simulink model "nexus_block"  (R2024b)
settings: Solver=ode4  StartTime=0.0  StopTime=5  FixedStep=0.001  RelTol=1e-3  AbsTol=1e-6
values from neighbouring files (symbols this model uses):
  Acf = [Acf zeros(3,3); zeros(3,3) Acf]    [nexus_fsm.m]
  Adc = [0 1 zeros(1,10); -wc^2 -2*zij(1,1)*wc zeros(1,10) ... (first row only)    [nexus_cryo.m]
  Adg = [Adg zeros(2,2); zeros(2,2) Adg]    [nexus_gs.m]
  Ads = [-wn]    [nexus_acsnoise.m]
  Adw = [Adr_r,zeros(4,8); zeros(4,4) Adr_a zeros(4,4); zeros(4,8) Adr_t]    [nexus_rwa.m]
  Bca = Bca*Tsel*[P' zeros(3,5); zeros(3,3) P' zeros(3,2); zeros(3,6) P'*H]    [nexus_acsloop.m]
  Bcf = [Bcf zeros(3,1); zeros(3,1) Bcf]    [nexus_fsm.m]
  Bdc = [0 1 0 1 0 1 0 1 0 1 0 1]'    [nexus_cryo.m]
  Bdg = [Bdg [0 0]';[0 0]' Bdg]    [nexus_gs.m]
  Bds = [1]'    [nexus_acsnoise.m]
  Bdw = [Bdr_r ; Bdr_a ; Bdr_t]    [nexus_rwa.m]
  Cca = (-1)*P*Cca    [nexus_acsloop.m]
  Ccf = [Ccf zeros(1,3); zeros(1,3) Ccf]    [nexus_fsm.m]
  Cdc = [       zeros(1,6) 0 kij(2,1) 0 kij(2,2) 0 kij(2,3) ... (first row only)    [nexus_cryo.m]
  Cdg = a2r*[Cdg [0 0]; [0 0] Cdg]    [nexus_gs.m]
  Cds = Kn*[wn]    [nexus_acsnoise.m]
  Cdw = [Cdr_r zeros(1,8); Cdr_r zeros(1,8); zeros(1,4) Cdr_a zeros(1,4) ... (first row only)    [nexus_rwa.m]
  Dca = (-1)*P*Dca*Tsel*[P' zeros(3,5); zeros(3,3) P' zeros(3,2); zeros(3,6) P'*H]    [nexus_acsloop.m]
  dcdu = inv(m2micron)*[dcdupmseg1 dcdupmseg2 dcdupmseg3 dcdusm dcduim]    [nexus_optics.m]
  Dcf = [Dcf 0; 0 Dcf]    [nexus_fsm.m]
  Ddc = [zeros(3,1)]    [nexus_cryo.m]
  Ddg = a2r*zeros(2,2)    [nexus_gs.m]
  Dds = [0]    [nexus_acsnoise.m]
  Ddw = [zeros(6,1)]    [nexus_rwa.m]
  dt = 1/(20*wc/2/pi)    [nexus_cryo.m]    (also in nexus_perf.m = 0.001)
  dwdu = inv(m2nm)*dwdu    [nexus_optics.m]    (also in nexus_perf.m = dwdu(1:nray,1:ndof))
  Kfsm = mm2m*dcdu(:,97:98)    [nexus_optics.m]
  m2micron = 1e6    (= 1000000)    [nexus_optics.m]
  m2nm = 1e9    (= 1000000000)    [nexus_optics.m]
  psc = mean(abs([sourcerot(1,1) sourcerot(2,2)]))    [nexus_optics.m]
  Seed = round(1e5*rand(10,1))    [nexus_perf.m]
undefined symbols (not defined in the file or in its folder): Aca, Ap, Bp, Cp, Dp, R1, R2, R3, R4
libraries: simulink x10, dspstat3 x2
settings Model: Creator=June  LastModifiedBy=June
settings SolverCC: AutoScaleAbsTol=off
settings DataIOCC: SaveFormat=Array  SignalLoggingSaveFormat=ModelDataLogs  ReturnWorkspaceOutputs=off
settings OptimizationCC: BlockReduction=off  BooleanDataType=off  ZeroExternalMemoryAtStartup=off  ZeroInternalMemoryAtStartup=off  InitFltsAndDblsToZero=on  LifeSpan=inf
settings DebuggingCC: SaveWithParameterizedLinksMsg=none  UnderspecifiedInitializationDetection=Classic  MergeDetectMultiDrivingBlocksExec=none  SignalResolutionControl=TryResolveAllWithWarning  MultiTaskDSMMsg=warning  MultiTaskCondExecSysMsg=none  FcnCallInpInsideContextMsg=warning  UnconnectedInputMsg=warning  UnconnectedOutputMsg=warning  UnconnectedLineMsg=warning  SFUnexpectedBacktrackingDiag=warning  SFNoUnconditionalDefaultTransitionDiag=warning  SFExecutionAtInitializationDiag=none  ArithmeticOperatorsInVariantConditions=warning
settings HardwareCC: ProdBitPerPointer=32  ProdBitPerSizeT=32  ProdBitPerPtrDiffT=32  ProdLargestAtomicFloat=None  ProdIntDivRoundTo=Undefined  ProdEndianess=Unspecified  ProdWordSize=32  ProdHWDeviceType=32-bit Generic  TargetBitPerPointer=64  TargetBitPerSizeT=64  TargetBitPerPtrDiffT=64  TargetLongLongMode=on  TargetIntDivRoundTo=Zero  TargetEndianess=LittleEndian  TargetWordSize=64  TargetHWDeviceType=MATLAB Host  ProdEqTarget=off
settings ModelReferenceCC: PropagateSignalLabelsOutOfModel=off
settings RTWCC: TargetLang=C++  GPUComputeCapability=3.5
settings CodeAppCC: ForceParamTrailComments=on  StateflowObjectComments=on  MATLABSourceComments=on
settings GRTTargetCC: TargetFcnLib=ansi_tfl_tmw.mat  TargetLangStandard=C++11 (ISO)  ModelReferenceCompliant=off  CodeInterfacePackaging=C++ class  MultiInstanceErrorCode=Warning
settings ConfigComp: CovMetricSettings=dw  CovSaveCumulativeToWorkspaceVar=on  CovSaveSingleToWorkspaceVar=on

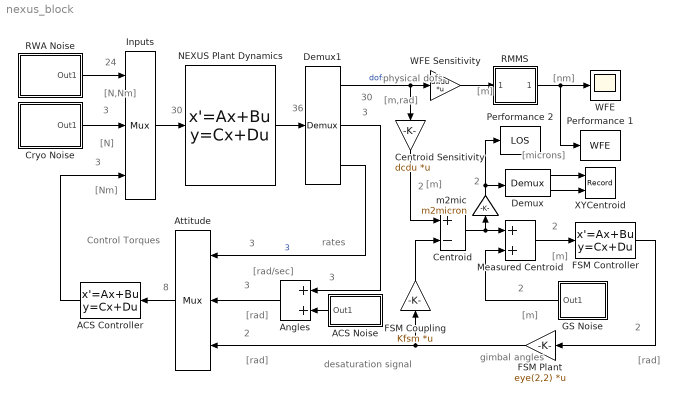
== system nexus_block ==
  note: 24
  note: 3
  note: 30
  note: 30
  note: 2
  note: 2
  note: 3
  note: 3
  note: 2
  note: 2
  note: gimbal
      | angles
  note: 36
  note: Control
      | Torques
  note: physical
      |  dofs
  note: rates
  note: 3
  note: 3
  note: 2
  note: 8
  note: desaturation signal
  note: [rad]
  note: [m,rad]
  note: [Nm]
  note: [rad/sec]
  note: [rad]
  note: [rad]
  note: [m]
  note: [m]
  note: [N,Nm]
  note: [N]
  note: [nm]
  note: [m]
  note: [microns]
  note: [m]
  note: 2
  note: 3
  ACS Controller : StateSpace  A=Aca  B=Bca  C=Cca  D=Dca  InitialCondition=0
  ACS Noise : Subsystem
  Angles : Sum  InputSameDT=on  SaturateOnIntegerOverflow=on  OutDataTypeStr=Inherit: Same as first input
  Attitude : Mux  Inputs=3
  Centroid : Sum  Inputs=+-  InputSameDT=on  SaturateOnIntegerOverflow=on  OutDataTypeStr=Inherit: Same as first input
  Centroid Sensitivity : Gain  Gain=dcdu  Multiplication=Matrix(K*u)  SaturateOnIntegerOverflow=on  OutDataTypeStr=Inherit: Same as input  ParamDataTypeStr=Inherit: Same as input
  Cryo Noise : Subsystem
  Demux : Demux  Outputs=2
      settings: DisplayOption=none
  Demux1 : Demux  Outputs=[30 3 3]
      settings: DisplayOption=none
  FSM Coupling : Gain  Gain=Kfsm  Multiplication=Matrix(K*u)  SaturateOnIntegerOverflow=on  OutDataTypeStr=Inherit: Same as input  ParamDataTypeStr=Inherit: Same as input
  FSM Controller : StateSpace  A=Acf  B=Bcf  C=(-1)*Ccf  D=(-1)*Dcf  InitialCondition=0
  FSM Plant : Gain  Gain=eye(2,2)  Multiplication=Matrix(K*u)  SaturateOnIntegerOverflow=on  OutDataTypeStr=Inherit: Same as input  ParamDataTypeStr=Inherit: Same as input
  GS Noise : Subsystem
  Inputs : Mux  Inputs=3
  Measured Centroid : Sum  InputSameDT=on  SaturateOnIntegerOverflow=on  OutDataTypeStr=Inherit: Same as first input
  NEXUS Plant Dynamics : StateSpace  A=Ap  B=Bp  C=Cp  D=Dp  InitialCondition=0
  Performance 1 : ToWorkspace  VariableName=WFE  SampleTime=dt
  Performance 2 : ToWorkspace  VariableName=LOS  SampleTime=-1
  RMMS : Subsystem
  RWA Noise : Subsystem
  WFE : Scope
  WFE Sensitivity : Gain  Gain=dwdu  Multiplication=Matrix(K*u)  SaturateOnIntegerOverflow=on  OutDataTypeStr=Inherit: Same as input  ParamDataTypeStr=Inherit: Same as input
  XYCentroid : Record  FileSettingsInternal="{\"entries\":[{\"content\":{\"excelSettings\":{\"content\":{},\"type\":\"Streamout.ExcelSettings\"}},\"type\":\"Streamout.FileSettingStorage\",\"uuid\":\"\"}],\"packageUris\":[\"http:\\/\\/schema.mathworks.com\\/mf0\\/streamout_blocks\\/R2020a\"],\"version\":\"1.0\"}"  Layout=[1 1]  SignalsInternal="{\"entries\":[{\"content\":{\"signals\":[{\"content\":{\"blockPath\":[],\"dimensions\":[1],\"domain\":\"\",\"lineColor\":\"#a2142f\",\"plots\":[ 1 ],\"port\":1,\"sid\":[\"\"],\"signalID\":1,\"signalName\":\"Demux:1\"},\"type\":\"RecordBlkView.Signal\",\"uuid\":\"\"},{\"content\":{\"blockPath\":[],\"dimensions\":[1],\"domain\":\"\",\"lineColor\":\"#139fff\",\"plots\":[ 1 ],\"port\":2,\"sid\":[\"\"],\"signalID\":2,\"signalName\":\"Demux:2\"},\"type\":\"RecordBlkView.Signal\",\"uuid\":\"\"}]},\"type\":\"RecordBlkView.InputSignals\",\"uuid\":\"\"}],\"packageUris\":[\"http:\\/\\/schema.mathworks.com\\/mf0\\/streamout_blocks\\/R2020a\"],\"version\":\"1.0\"}"  VisualizationBindings="{\"xyplotplugin\":{\"info\":[{\"series\":[{\"bindingParametersList\":[{\"parameter\":\"X-Axis\",\"signalID\":1,\"signalName\":\"Demux:1\"},{\"parameter\":\"Y-Axis\",\"signalID\":2,\"signalName\":\"Demux:2\"}],\"seriesID\":0}],\"subplotID\":1}]}}"  CompatibilityTag=XY  st=dt
  m2mic : Gain  Gain=m2micron  SaturateOnIntegerOverflow=on  OutDataTypeStr=Inherit: Same as input  ParamDataTypeStr=Inherit: Same as input
  wires:
  Inputs/1 -> NEXUS Plant Dynamics/1
  NEXUS Plant Dynamics/1 -> Demux1/1
  ACS Controller/1 -> Inputs/3
  Attitude/1 -> ACS Controller/1
  Angles/1 -> Attitude/2
  Demux1/2 -> Angles/1
  Demux1/1 -> WFE Sensitivity/1, Centroid Sensitivity/1  "dofs"
  Centroid Sensitivity/1 -> Centroid/1
  GS Noise/1(Out1) -> Measured Centroid/2
  Measured Centroid/1 -> FSM Controller/1
  ACS Noise/1(Out1) -> Angles/2
  FSM Coupling/1 -> Centroid/2
  RWA Noise/1(Out1) -> Inputs/1
  Cryo Noise/1(Out1) -> Inputs/2
  Demux1/3 -> Attitude/1  "3"
  Demux/1 -> XYCentroid/1
  Demux/2 -> XYCentroid/2
  FSM Controller/1 -> FSM Plant/1
  FSM Plant/1 -> Attitude/3, FSM Coupling/1
  RMMS/1(Out1) -> Performance 1/1, WFE/1
  Centroid/1 -> Measured Centroid/1, m2mic/1
  m2mic/1 -> Performance 2/1, Demux/1
  WFE Sensitivity/1 -> RMMS/1(In1)

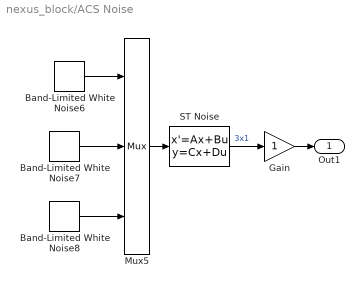
== system nexus_block/ACS Noise ==
  Band-Limited White Noise6 : simulink/Sources/Band-Limited White Noise  Cov=[1.0]  Ts=dt  seed=Seed(6)
  Band-Limited White Noise7 : simulink/Sources/Band-Limited White Noise  Cov=[1.0]  Ts=dt  seed=Seed(7)
  Band-Limited White Noise8 : simulink/Sources/Band-Limited White Noise  Cov=[1.0]  Ts=dt  seed=Seed(8)
  Gain : Gain  SaturateOnIntegerOverflow=on  OutDataTypeStr=Inherit: Same as input  ParamDataTypeStr=Inherit: Same as input
  Mux5 : Mux  Inputs=3
  ST Noise : StateSpace  A=Ads  B=Bds  C=Cds  D=Dds  InitialCondition=0
  Out1 : Outport
  wires:
  Band-Limited White Noise6/1 -> Mux5/1
  Band-Limited White Noise7/1 -> Mux5/2
  Band-Limited White Noise8/1 -> Mux5/3
  Mux5/1 -> ST Noise/1
  Gain/1 -> Out1/1
  ST Noise/1 -> Gain/1  "3x1"

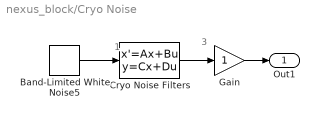
== system nexus_block/Cryo Noise ==
  note: 3
  note: 1
  Band-Limited White Noise5 : simulink/Sources/Band-Limited White Noise  Cov=[1.0]  Ts=dt  seed=Seed(5)
  Cryo Noise Filters : StateSpace  A=Adc  B=Bdc  C=Cdc  D=Ddc  InitialCondition=0
  Gain : Gain  SaturateOnIntegerOverflow=on  OutDataTypeStr=Inherit: Same as input  ParamDataTypeStr=Inherit: Same as input
  Out1 : Outport
  wires:
  Band-Limited White Noise5/1 -> Cryo Noise Filters/1
  Cryo Noise Filters/1 -> Gain/1
  Gain/1 -> Out1/1

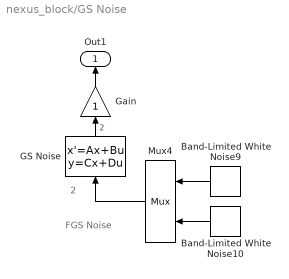
== system nexus_block/GS Noise ==
  note: FGS Noise
  note: 2
  Band-Limited White Noise10 : simulink/Sources/Band-Limited White Noise  Cov=[1.0]  Ts=dt  seed=Seed(10)
  Band-Limited White Noise9 : simulink/Sources/Band-Limited White Noise  Cov=[1.0]  Ts=dt  seed=Seed(9)
  GS Noise : StateSpace  A=Adg  B=Bdg  C=psc*Cdg  D=psc*Ddg  InitialCondition=0
  Gain : Gain  SaturateOnIntegerOverflow=on  OutDataTypeStr=Inherit: Same as input  ParamDataTypeStr=Inherit: Same as input
  Mux4 : Mux  Inputs=2
  Out1 : Outport
  wires:
  Mux4/1 -> GS Noise/1
  Band-Limited White Noise9/1 -> Mux4/1
  Band-Limited White Noise10/1 -> Mux4/2
  Gain/1 -> Out1/1
  GS Noise/1 -> Gain/1  "2"

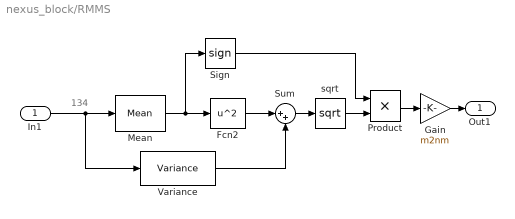
== system nexus_block/RMMS ==
  note: 134
  In1 : Inport
  Fcn2 : Fcn  Expr=u^2
  Gain : Gain  Gain=m2nm  SaturateOnIntegerOverflow=on  OutDataTypeStr=Inherit: Same as input  ParamDataTypeStr=Inherit: Same as input
  Mean : dspstat3/Mean  run=off  InputProcessing=Columns as channels (frame based)  reset_popup=None  directionMode=Each column  dimension=1  roiEnable=off  roiType=Rectangles  roiPortion=Entire ROI  roiOutput=Individual statistics for each ROI  roiFlag=off  roundingMode=Floor  overflowMode=off  outputDataTypeStr=Inherit: Same as accumulator  outputMin=[]  outputMax=[]  outputLastDataTypeStr=Inherit: Same as accumulator
  Product : Product  InputSameDT=on  RndMeth=Zero  SaturateOnIntegerOverflow=on  OutDataTypeStr=Inherit: Same as first input
  Sign : Signum
  Sum : Sum  Inputs=|++  InputSameDT=on  SaturateOnIntegerOverflow=on  OutDataTypeStr=Inherit: Same as first input
  Variance : dspstat3/Variance  run=off  InputProcessing=Columns as channels (frame based)  reset_popup=None  directionMode=Each column  dimension=1  roiEnable=off  roiType=Rectangles  roiPortion=Entire ROI  roiOutput=Individual statistics for each ROI  roiFlag=off  roundingMode=Floor  overflowMode=off
  sqrt : Math  Operator=sqrt  SignedPower=on
  Out1 : Outport
  wires:
  In1/1 -> Mean/1, Variance/1
  Mean/1 -> Fcn2/1, Sign/1
  Fcn2/1 -> Sum/1
  Variance/1 -> Sum/2
  Sum/1 -> sqrt/1
  sqrt/1 -> Product/2
  Sign/1 -> Product/1
  Product/1 -> Gain/1
  Gain/1 -> Out1/1

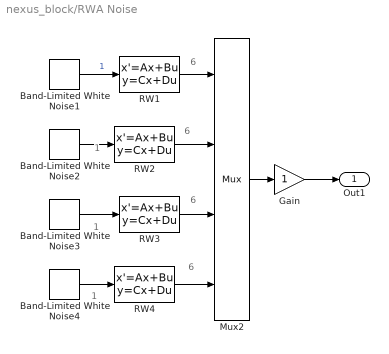
== system nexus_block/RWA Noise ==
  note: 1
  note: 1
  note: 1
  note: 6
  note: 6
  note: 6
  note: 6
  Band-Limited White Noise1 : simulink/Sources/Band-Limited White Noise  Cov=[1.0]  Ts=dt  seed=Seed(1)
  Band-Limited White Noise2 : simulink/Sources/Band-Limited White Noise  Cov=[1.0]  Ts=dt  seed=Seed(2)
  Band-Limited White Noise3 : simulink/Sources/Band-Limited White Noise  Cov=[1.0]  Ts=dt  seed=Seed(3)
  Band-Limited White Noise4 : simulink/Sources/Band-Limited White Noise  Cov=[1.0]  Ts=dt  seed=Seed(4)
  Gain : Gain  SaturateOnIntegerOverflow=on  OutDataTypeStr=Inherit: Same as input  ParamDataTypeStr=Inherit: Same as input
  Mux2 : Mux
  RW1 : StateSpace  A=Adw  B=Bdw  C=R1*Cdw  D=R1*Ddw  InitialCondition=0
  RW2 : StateSpace  A=Adw  B=Bdw  C=R2*Cdw  D=R2*Ddw  InitialCondition=0
  RW3 : StateSpace  A=Adw  B=Bdw  C=R3*Cdw  D=R3*Ddw  InitialCondition=0
  RW4 : StateSpace  A=Adw  B=Bdw  C=R4*Cdw  D=R4*Ddw  InitialCondition=0
  Out1 : Outport
  wires:
  Band-Limited White Noise1/1 -> RW1/1  "1"
  Band-Limited White Noise3/1 -> RW3/1
  Band-Limited White Noise4/1 -> RW4/1
  RW1/1 -> Mux2/1
  RW2/1 -> Mux2/2
  RW3/1 -> Mux2/3
  RW4/1 -> Mux2/4
  Band-Limited White Noise2/1 -> RW2/1
  Mux2/1 -> Gain/1
  Gain/1 -> Out1/1
